simulink model "Copy_of_AUV_main"  (R2020b)
settings: Solver=VariableStepAuto  StartTime=0.0  StopTime=400  FixedStep=0.1  RelTol=1e-3
libraries: pid_lib x4, robotcorelib x2, dspsigops x1
settings Model: Creator=shanerutherford  LastModifiedBy=shanerutherford
settings SolverCC: ZeroCrossAlgorithm=Adaptive
settings DebuggingCC: IgnoredZcDiagnostic=none

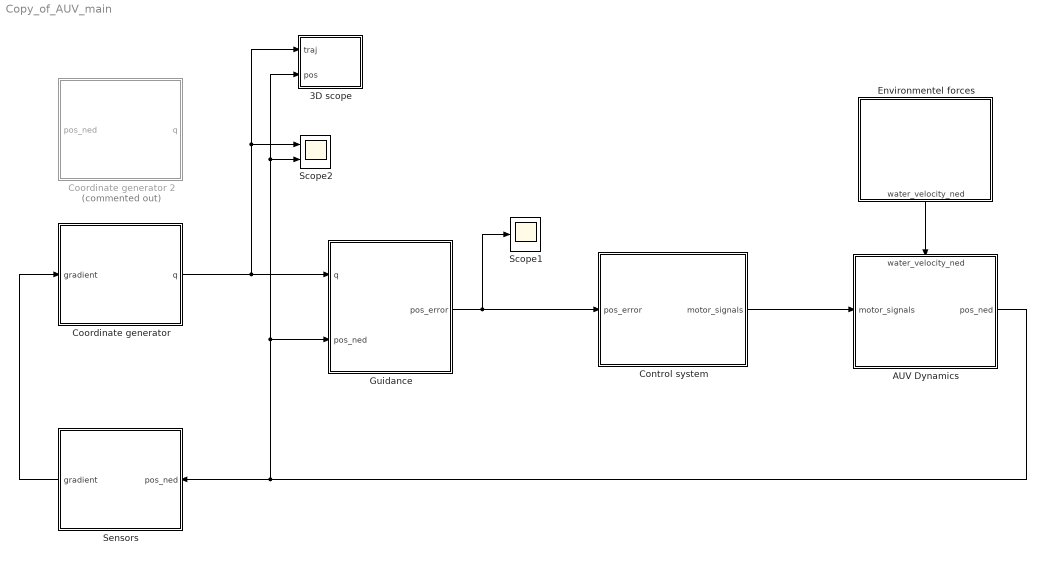
== system Copy_of_AUV_main ==
  3D scope : Subsystem
  AUV Dynamics : Subsystem
      settings: PortSchema="{\"entries\":[{\"content\":{\"sides\":[{\"content\":{\"connectorIds\":[\"In1\"]},\"type\":\"ConnectorPlacement.EquallySpacedRectSide\",\"uuid\":\"9ee444f3-b955-488d-8e49-640ea0f7df37\"},{\"content\":{\"connectorIds\":[\"Out1\"],\"side\":\"RIGHT\"},\"type\":\"ConnectorPlacement.EquallySpacedRectSide\",\"uuid\":\"ce4b5243-31e8-415d-aaa8-03cbb0c8065f\"},{\"content\":{\"connectorIds\":[\"In2\"],\"side\":\"TOP\"},\"type\":\"ConnectorPlacement.EquallySpacedRectSide\",\"uuid\":\"f69ed04b-67fd-4237-ab1a-d9f9564e83a0\"},{\"content\":{\"connectorIds\":[],\"side\":\"HIDDEN\"},\"type\":\"ConnectorPlacement.EquallySpacedRectSide\",\"uuid\":\"5b6b6d1e-b1c4-449c-9873-97d05fa29e3c\"}]},\"type\":\"ConnectorPlacement.EquallySpacedConnector\",\"uuid\":\"e4d51cd1-1a50-495c-8222-c38a5b01ba84\"}],\"packageUris\":[\"http://schema.mathworks.com/mf0/Connector/R2020b\"],\"version\":\"1.0\"}"
  Control system : Subsystem
  Coordinate generator : Subsystem
  Coordinate generator 2 : Subsystem  Commented=on
  Environmentel forces : Subsystem
      settings: PortSchema="{\"entries\":[{\"content\":{\"sides\":[{\"content\":{\"connectorIds\":[]},\"type\":\"ConnectorPlacement.EquallySpacedRectSide\",\"uuid\":\"0dd98e89-aff4-433c-b28f-c29455b8a07d\"},{\"content\":{\"connectorIds\":[],\"side\":\"RIGHT\"},\"type\":\"ConnectorPlacement.EquallySpacedRectSide\",\"uuid\":\"953662a4-5b51-4456-b69c-eca28c97a39b\"},{\"content\":{\"connectorIds\":[],\"side\":\"TOP\"},\"type\":\"ConnectorPlacement.EquallySpacedRectSide\",\"uuid\":\"911274c2-620a-4054-9b06-c69233cda7b5\"},{\"content\":{\"connectorIds\":[\"Out1\"],\"side\":\"BOTTOM\"},\"type\":\"ConnectorPlacement.EquallySpacedRectSide\",\"uuid\":\"d1098ec8-c176-4eae-9d99-8b466f13cb7d\"},{\"content\":{\"connectorIds\":[],\"side\":\"HIDDEN\"},\"type\":\"ConnectorPlacement.EquallySpacedRectSide\",\"uuid\":\"331d0c74-f854-4ce9-a20e-6d7219b69b25\"}]},\"type\":\"ConnectorPlacement.EquallySpacedConnector\",\"uuid\":\"51f6c218-3b35-4d9f-b9df-5dfda31bafc0\"}],\"packageUris\":[\"http://schema.mathworks.com/mf0/Connector/R2020b\"],\"version\":\"1.0\"}"
  Guidance : Subsystem
  Scope1 : Scope
  Scope2 : Scope  NumInputPorts=2
  Sensors : Subsystem
  wires:
  Guidance/1(pos_error) -> Control system/1(pos_error), Scope1/1
  AUV Dynamics/1(pos_ned) -> Sensors/1(pos_ned), 3D scope/2(pos), Scope2/2, Guidance/2(pos_ned)
  Environmentel forces/1(water_velocity_ned) -> AUV Dynamics/2(water_velocity_ned)
  Control system/1(motor_signals) -> AUV Dynamics/1(motor_signals)
  Coordinate generator/1(q) -> 3D scope/1(traj), Scope2/1, Guidance/1(q)
  Sensors/1(gradient) -> Coordinate generator/1(gradient)

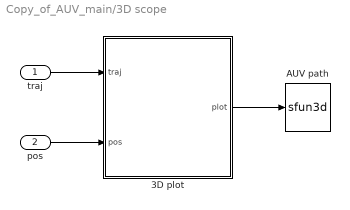
== system Copy_of_AUV_main/3D scope ==
  traj : Inport
  pos : Inport  Port=2
  3D plot : MATLAB Function  TreatAsAtomicUnit=on
  AUV path : S-Function  LoadFcn=if exist('sfun3d','file'), sfun3d([],[],[],'LoadBlock'); end  FunctionName=sfun3d  Parameters=ax,T,np,cp,gd,ls,mk,mx,hd,tb  SFunctionDeploymentMode=off  EnableBusSupport=off  mask(3D Graph){np=2, ax=[-15 15 -15 15 -20 20], mx=1e4, T=-1, cp=[0, 0 15], gd=on, hd=on, tb=on, ls=-, mk=none}
      mask prompts: np "Number of moving points (lines)"; ax "Range: [xmin xmax  ymin ymax zmin zmax]"; mx "Max number of points in each line"; T "Sampling Time"; cp "Camera position (use [0 0 1] for 2D XY view)"; gd "Grid (on|off)"; hd "HeadMarkers (on|off)"; tb "Toolbar (on|off)"; ls "LineStyle"; mk "LineMarker"
      mask help:
      | This block plots the position of several points in the XYZ space. The input contains the coordinates of all the points (x1,y1,z1,x2,y2,z2,...).
      | The number of moving points (lines), the XYZ ranges, sampling time, camera position, and grid (among other things) can be set as mask parameters.
      settings: CopyFcn=if exist('sfun3d','file'), sfun3d([],[],[],'CopyBlock'); end  DeleteFcn=if exist('sfun3d','file'), sfun3d([],[],[],'DeleteBlock'); end  NameChangeFcn=if exist('sfun3d','file'), sfun3d([],[],[],'NameChange'); end
      mask Help:
      | This block plots the position of several points in the XYZ space. The input contains the coordinates of all the points (x1,y1,z1,x2,y2,z2,...).
      | The number of moving points (lines), the XYZ ranges, sampling time, camera position, and grid (among other things) can be set as mask parameters.
      mask TypeOptions ls: - | -- | : | -. | none
      mask TypeOptions mk: none | . | + | o | * | x | square | diamond | v | ^ | > | < | pentagram | hexagram
      mask Display: plot([.05 .95 .95 .05 .05],[.45 .45 .95 .95 .45], 0.5+cos(0:0.1:2*pi)*0.3,0.7+sin(0:0.1:2*pi)*0.2)
  wires:
  3D plot/1(plot) -> AUV path/1
  traj/1 -> 3D plot/1(traj)
  pos/1 -> 3D plot/2(pos)

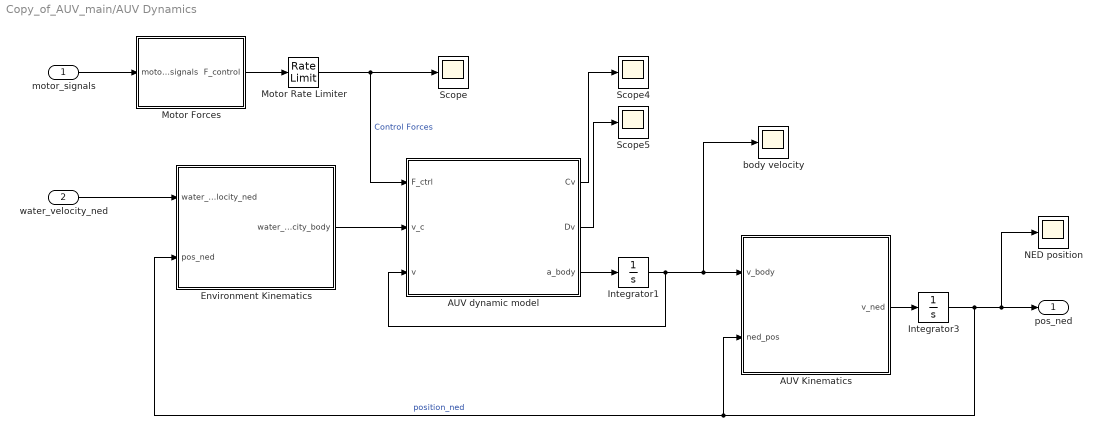
== system Copy_of_AUV_main/AUV Dynamics ==
  motor_signals : Inport
  water_velocity_ned : Inport  Port=2
  AUV Kinematics : MATLAB Function  TreatAsAtomicUnit=on
  AUV dynamic model : MATLAB Function  TreatAsAtomicUnit=on
  Environment Kinematics : MATLAB Function  TreatAsAtomicUnit=on
  Integrator1 : Integrator
  Integrator3 : Integrator
  Motor Forces : MATLAB Function  TreatAsAtomicUnit=on
  Motor Rate Limiter : RateLimiter  RisingSlewLimit=10  FallingSlewLimit=-10  SampleTimeMode=inherited
  NED position : Scope
  Scope : Scope
  Scope4 : Scope
  Scope5 : Scope
  body velocity : Scope
  pos_ned : Outport  PortDimensions=6
  wires:
  Integrator3/1 -> pos_ned/1, NED position/1, Environment Kinematics/2(pos_ned), AUV Kinematics/2(ned_pos)  "position_ned"
  Environment Kinematics/1(water_velocity_body) -> AUV dynamic model/2(v_c)
  AUV dynamic model/3(a_body) -> Integrator1/1
  AUV Kinematics/1(v_ned) -> Integrator3/1
  AUV dynamic model/1(Cv) -> Scope4/1
  Integrator1/1 -> AUV Kinematics/1(v_body), body velocity/1, AUV dynamic model/3(v)
  AUV dynamic model/2(Dv) -> Scope5/1
  water_velocity_ned/1 -> Environment Kinematics/1(water_velocity_ned)
  Motor Forces/1(F_control) -> Motor Rate Limiter/1
  motor_signals/1 -> Motor Forces/1(motor_signals)
  Motor Rate Limiter/1 -> AUV dynamic model/1(F_ctrl), Scope/1  "Control Forces"

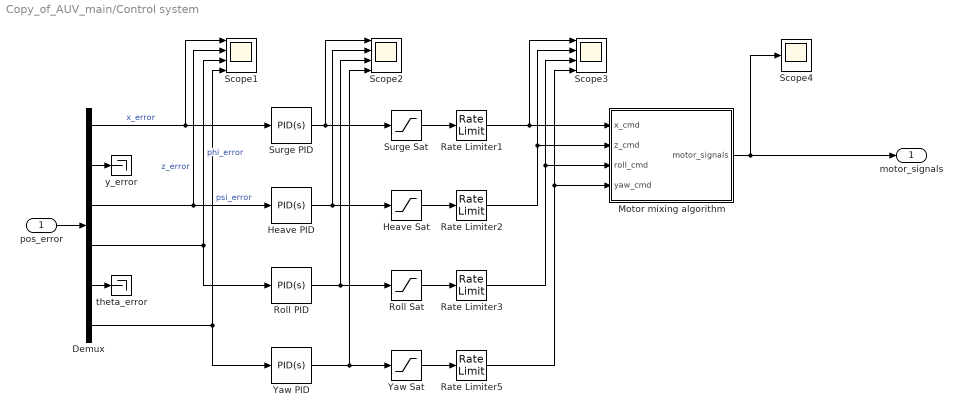
== system Copy_of_AUV_main/Control system ==
  pos_error : Inport
  Demux : Demux  Outputs=6
  Heave PID : pid_lib/PID Controller  Controller=PID  Form=Parallel  TimeDomain=Continuous-time  UseExternalTs=off  SampleTime=-1  IntegratorMethod=Forward Euler  FilterMethod=Forward Euler  ControllerParametersSource=internal  P=10  I=0  D=5  UseFilter=on  N=100  TunerSelectOption=Transfer Function Based (PID Tuner App)  InitialConditionSource=internal  InitialConditionForIntegrator=0  InitialConditionForFilter=0  DifferentiatorICPrevScaledInput=0  ExternalReset=none  TrackingMode=off  Kt=1  LimitOutput=on  SatLimitsSource=internal  UpperSaturationLimit=100  LowerSaturationLimit=-100  LinearizeAsGain=on  AntiWindupMode=none  Kb=1  POutMin=[]  POutMax=[]  IOutMin=[]  IOutMax=[]  DOutMin=[]  DOutMax=[]  NOutMin=[]  NOutMax=[]  SumOutMin=[]  SumOutMax=[]  SaturationOutMin=[]  SaturationOutMax=[]  PParamMin=[]  PParamMax=[]  IParamMin=[]  IParamMax=[]  DParamMin=[]  DParamMax=[]  NParamMin=[]  NParamMax=[]  KbParamMin=[]  KbParamMax=[]  KtParamMin=[]  KtParamMax=[]  KbOutMin=[]  KbOutMax=[]  KtOutMin=[]  KtOutMax=[]  IntegratorOutMin=[]  IntegratorOutMax=[]  FilterOutMin=[]  FilterOutMax=[]  SumI1OutMin=[]  SumI1OutMax=[]  SumI2OutMin=[]  SumI2OutMax=[]  SumI3OutMin=[]  SumI3OutMax=[]  SumI4OutMin=[]  SumI4OutMax=[]  SumDOutMin=[]  SumDOutMax=[]  DifferentiatorOutMin=[]  DifferentiatorOutMax=[]  FilterDiffOutCoefMin=[]  FilterDiffOutCoefMax=[]  ReciprocalOutMin=[]  ReciprocalOutMax=[]  SumDenOutMin=[]  SumDenOutMax=[]  SumNumOutMin=[]  SumNumOutMax=[]  DivideOutMin=[]  DivideOutMax=[]  UdiffTsProdOutMin=[]  UdiffTsProdOutMax=[]  NTsProdOutMin=[]  NTsProdOutMax=[]  UintegralTsProdOutMin=[]  UintegralTsProdOutMax=[]  UngainTsProdOutMin=[]  UngainTsProdOutMax=[]  IntegratorContinuousStateAttributes=''  IntegratorStateMustResolveToSignalObject=off  IntegratorRTWStateStorageClass=Auto  FilterContinuousStateAttributes=''  FilterStateMustResolveToSignalObject=off  FilterRTWStateStorageClass=Auto  ParallelPVariant=InternalParameters  IdealPVariant=Disabled  IVariant=InternalParameters  DVariant=InternalParameters  IntegratorVariant=Continuous  SatVariant=Enabled  AWVariant=Passthrough  PCopyVariant=Disabled  TRVariant=Disabled  FdbkBlocksVariant=Forward  IdealPFdbkVariant=Disabled  SatFdbkVariant=Disabled  DerivativeFilterVariant=ContFilter  NVariant=InternalParameters  NCopyVariant=Disabled  FilterICVariant=InternalICsFilter  IntegratorICVariant=InternalICs  ExternalResetVariant=Disabled  TRSumVariant=Passthrough  SumFdbkVariant=Disabled  SumVariant=Sum_PID  TsampFilterVariant=InternalTs  TsampNgainVariant=Passthrough  TsampIntegralVariant=Passthrough  ExternalSaturationOutDataTypeStr=Inherit: Same as second input
  Heave Sat : Saturate  UpperLimit=40  LowerLimit=-40  ZeroCross=off
  Motor mixing algorithm : MATLAB Function  TreatAsAtomicUnit=on
  Rate Limiter{1..3,5} (4 alike) : RateLimiter  RisingSlewLimit=20  FallingSlewLimit=-20  SampleTimeMode=inherited
  Roll PID : pid_lib/PID Controller  Controller=PID  Form=Parallel  TimeDomain=Continuous-time  UseExternalTs=off  SampleTime=-1  IntegratorMethod=Forward Euler  FilterMethod=Forward Euler  ControllerParametersSource=internal  P=20  I=0  D=10  UseFilter=on  N=100  TunerSelectOption=Transfer Function Based (PID Tuner App)  InitialConditionSource=internal  InitialConditionForIntegrator=0  InitialConditionForFilter=0  DifferentiatorICPrevScaledInput=0  ExternalReset=none  TrackingMode=off  Kt=1  LimitOutput=on  SatLimitsSource=internal  UpperSaturationLimit=100  LowerSaturationLimit=-100  LinearizeAsGain=on  AntiWindupMode=none  Kb=1  POutMin=[]  POutMax=[]  IOutMin=[]  IOutMax=[]  DOutMin=[]  DOutMax=[]  NOutMin=[]  NOutMax=[]  SumOutMin=[]  SumOutMax=[]  SaturationOutMin=[]  SaturationOutMax=[]  PParamMin=[]  PParamMax=[]  IParamMin=[]  IParamMax=[]  DParamMin=[]  DParamMax=[]  NParamMin=[]  NParamMax=[]  KbParamMin=[]  KbParamMax=[]  KtParamMin=[]  KtParamMax=[]  KbOutMin=[]  KbOutMax=[]  KtOutMin=[]  KtOutMax=[]  IntegratorOutMin=[]  IntegratorOutMax=[]  FilterOutMin=[]  FilterOutMax=[]  SumI1OutMin=[]  SumI1OutMax=[]  SumI2OutMin=[]  SumI2OutMax=[]  SumI3OutMin=[]  SumI3OutMax=[]  SumI4OutMin=[]  SumI4OutMax=[]  SumDOutMin=[]  SumDOutMax=[]  DifferentiatorOutMin=[]  DifferentiatorOutMax=[]  FilterDiffOutCoefMin=[]  FilterDiffOutCoefMax=[]  ReciprocalOutMin=[]  ReciprocalOutMax=[]  SumDenOutMin=[]  SumDenOutMax=[]  SumNumOutMin=[]  SumNumOutMax=[]  DivideOutMin=[]  DivideOutMax=[]  UdiffTsProdOutMin=[]  UdiffTsProdOutMax=[]  NTsProdOutMin=[]  NTsProdOutMax=[]  UintegralTsProdOutMin=[]  UintegralTsProdOutMax=[]  UngainTsProdOutMin=[]  UngainTsProdOutMax=[]  IntegratorContinuousStateAttributes=''  IntegratorStateMustResolveToSignalObject=off  IntegratorRTWStateStorageClass=Auto  FilterContinuousStateAttributes=''  FilterStateMustResolveToSignalObject=off  FilterRTWStateStorageClass=Auto  ParallelPVariant=InternalParameters  IdealPVariant=Disabled  IVariant=InternalParameters  DVariant=InternalParameters  IntegratorVariant=Continuous  SatVariant=Enabled  AWVariant=Passthrough  PCopyVariant=Disabled  TRVariant=Disabled  FdbkBlocksVariant=Forward  IdealPFdbkVariant=Disabled  SatFdbkVariant=Disabled  DerivativeFilterVariant=ContFilter  NVariant=InternalParameters  NCopyVariant=Disabled  FilterICVariant=InternalICsFilter  IntegratorICVariant=InternalICs  ExternalResetVariant=Disabled  TRSumVariant=Passthrough  SumFdbkVariant=Disabled  SumVariant=Sum_PID  TsampFilterVariant=InternalTs  TsampNgainVariant=Passthrough  TsampIntegralVariant=Passthrough  ExternalSaturationOutDataTypeStr=Inherit: Same as second input
  Roll Sat : Saturate  UpperLimit=40  LowerLimit=-40  ZeroCross=off
  Scope1 : Scope  NumInputPorts=4
  Scope2 : Scope  NumInputPorts=4
  Scope3 : Scope  NumInputPorts=4
  Scope4 : Scope
  Surge PID : pid_lib/PID Controller  Controller=PID  Form=Parallel  TimeDomain=Continuous-time  UseExternalTs=off  SampleTime=-1  IntegratorMethod=Forward Euler  FilterMethod=Forward Euler  ControllerParametersSource=internal  P=10  I=0  D=5  UseFilter=on  N=100  TunerSelectOption=Transfer Function Based (PID Tuner App)  InitialConditionSource=internal  InitialConditionForIntegrator=0  InitialConditionForFilter=0  DifferentiatorICPrevScaledInput=0  ExternalReset=none  TrackingMode=off  Kt=1  LimitOutput=on  SatLimitsSource=internal  UpperSaturationLimit=100  LowerSaturationLimit=-100  LinearizeAsGain=on  AntiWindupMode=none  Kb=1  POutMin=[]  POutMax=[]  IOutMin=[]  IOutMax=[]  DOutMin=[]  DOutMax=[]  NOutMin=[]  NOutMax=[]  SumOutMin=[]  SumOutMax=[]  SaturationOutMin=[]  SaturationOutMax=[]  PParamMin=[]  PParamMax=[]  IParamMin=[]  IParamMax=[]  DParamMin=[]  DParamMax=[]  NParamMin=[]  NParamMax=[]  KbParamMin=[]  KbParamMax=[]  KtParamMin=[]  KtParamMax=[]  KbOutMin=[]  KbOutMax=[]  KtOutMin=[]  KtOutMax=[]  IntegratorOutMin=[]  IntegratorOutMax=[]  FilterOutMin=[]  FilterOutMax=[]  SumI1OutMin=[]  SumI1OutMax=[]  SumI2OutMin=[]  SumI2OutMax=[]  SumI3OutMin=[]  SumI3OutMax=[]  SumI4OutMin=[]  SumI4OutMax=[]  SumDOutMin=[]  SumDOutMax=[]  DifferentiatorOutMin=[]  DifferentiatorOutMax=[]  FilterDiffOutCoefMin=[]  FilterDiffOutCoefMax=[]  ReciprocalOutMin=[]  ReciprocalOutMax=[]  SumDenOutMin=[]  SumDenOutMax=[]  SumNumOutMin=[]  SumNumOutMax=[]  DivideOutMin=[]  DivideOutMax=[]  UdiffTsProdOutMin=[]  UdiffTsProdOutMax=[]  NTsProdOutMin=[]  NTsProdOutMax=[]  UintegralTsProdOutMin=[]  UintegralTsProdOutMax=[]  UngainTsProdOutMin=[]  UngainTsProdOutMax=[]  IntegratorContinuousStateAttributes=''  IntegratorStateMustResolveToSignalObject=off  IntegratorRTWStateStorageClass=Auto  FilterContinuousStateAttributes=''  FilterStateMustResolveToSignalObject=off  FilterRTWStateStorageClass=Auto  ParallelPVariant=InternalParameters  IdealPVariant=Disabled  IVariant=InternalParameters  DVariant=InternalParameters  IntegratorVariant=Continuous  SatVariant=Enabled  AWVariant=Passthrough  PCopyVariant=Disabled  TRVariant=Disabled  FdbkBlocksVariant=Forward  IdealPFdbkVariant=Disabled  SatFdbkVariant=Disabled  DerivativeFilterVariant=ContFilter  NVariant=InternalParameters  NCopyVariant=Disabled  FilterICVariant=InternalICsFilter  IntegratorICVariant=InternalICs  ExternalResetVariant=Disabled  TRSumVariant=Passthrough  SumFdbkVariant=Disabled  SumVariant=Sum_PID  TsampFilterVariant=InternalTs  TsampNgainVariant=Passthrough  TsampIntegralVariant=Passthrough  ExternalSaturationOutDataTypeStr=Inherit: Same as second input
  Surge Sat : Saturate  UpperLimit=40  LowerLimit=-40  ZeroCross=off
  Yaw PID : pid_lib/PID Controller  Controller=PID  Form=Parallel  TimeDomain=Continuous-time  UseExternalTs=off  SampleTime=-1  IntegratorMethod=Forward Euler  FilterMethod=Forward Euler  ControllerParametersSource=internal  P=20  I=0  D=10  UseFilter=on  N=100  TunerSelectOption=Transfer Function Based (PID Tuner App)  InitialConditionSource=internal  InitialConditionForIntegrator=0  InitialConditionForFilter=0  DifferentiatorICPrevScaledInput=0  ExternalReset=none  TrackingMode=off  Kt=1  LimitOutput=on  SatLimitsSource=internal  UpperSaturationLimit=100  LowerSaturationLimit=-100  LinearizeAsGain=on  AntiWindupMode=none  Kb=1  POutMin=[]  POutMax=[]  IOutMin=[]  IOutMax=[]  DOutMin=[]  DOutMax=[]  NOutMin=[]  NOutMax=[]  SumOutMin=[]  SumOutMax=[]  SaturationOutMin=[]  SaturationOutMax=[]  PParamMin=[]  PParamMax=[]  IParamMin=[]  IParamMax=[]  DParamMin=[]  DParamMax=[]  NParamMin=[]  NParamMax=[]  KbParamMin=[]  KbParamMax=[]  KtParamMin=[]  KtParamMax=[]  KbOutMin=[]  KbOutMax=[]  KtOutMin=[]  KtOutMax=[]  IntegratorOutMin=[]  IntegratorOutMax=[]  FilterOutMin=[]  FilterOutMax=[]  SumI1OutMin=[]  SumI1OutMax=[]  SumI2OutMin=[]  SumI2OutMax=[]  SumI3OutMin=[]  SumI3OutMax=[]  SumI4OutMin=[]  SumI4OutMax=[]  SumDOutMin=[]  SumDOutMax=[]  DifferentiatorOutMin=[]  DifferentiatorOutMax=[]  FilterDiffOutCoefMin=[]  FilterDiffOutCoefMax=[]  ReciprocalOutMin=[]  ReciprocalOutMax=[]  SumDenOutMin=[]  SumDenOutMax=[]  SumNumOutMin=[]  SumNumOutMax=[]  DivideOutMin=[]  DivideOutMax=[]  UdiffTsProdOutMin=[]  UdiffTsProdOutMax=[]  NTsProdOutMin=[]  NTsProdOutMax=[]  UintegralTsProdOutMin=[]  UintegralTsProdOutMax=[]  UngainTsProdOutMin=[]  UngainTsProdOutMax=[]  IntegratorContinuousStateAttributes=''  IntegratorStateMustResolveToSignalObject=off  IntegratorRTWStateStorageClass=Auto  FilterContinuousStateAttributes=''  FilterStateMustResolveToSignalObject=off  FilterRTWStateStorageClass=Auto  ParallelPVariant=InternalParameters  IdealPVariant=Disabled  IVariant=InternalParameters  DVariant=InternalParameters  IntegratorVariant=Continuous  SatVariant=Enabled  AWVariant=Passthrough  PCopyVariant=Disabled  TRVariant=Disabled  FdbkBlocksVariant=Forward  IdealPFdbkVariant=Disabled  SatFdbkVariant=Disabled  DerivativeFilterVariant=ContFilter  NVariant=InternalParameters  NCopyVariant=Disabled  FilterICVariant=InternalICsFilter  IntegratorICVariant=InternalICs  ExternalResetVariant=Disabled  TRSumVariant=Passthrough  SumFdbkVariant=Disabled  SumVariant=Sum_PID  TsampFilterVariant=InternalTs  TsampNgainVariant=Passthrough  TsampIntegralVariant=Passthrough  ExternalSaturationOutDataTypeStr=Inherit: Same as second input
  Yaw Sat : Saturate  UpperLimit=40  LowerLimit=-40  ZeroCross=off
  theta_error : Terminator
  y_error : Terminator
  motor_signals : Outport
  wires:
  Demux/4 -> Scope1/3, Roll PID/1  "phi_error"
  Surge Sat/1 -> Rate Limiter1/1
  Demux/3 -> Scope1/2, Heave PID/1  "z_error"
  Roll Sat/1 -> Rate Limiter3/1
  Demux/6 -> Scope1/4, Yaw PID/1  "psi_error"
  Yaw Sat/1 -> Rate Limiter5/1
  Heave Sat/1 -> Rate Limiter2/1
  Demux/1 -> Scope1/1, Surge PID/1  "x_error"
  pos_error/1 -> Demux/1
  Demux/5 -> theta_error/1
  Demux/2 -> y_error/1
  Yaw PID/1 -> Scope2/4, Yaw Sat/1
  Roll PID/1 -> Roll Sat/1, Scope2/3
  Heave PID/1 -> Heave Sat/1, Scope2/2
  Surge PID/1 -> Surge Sat/1, Scope2/1
  Rate Limiter1/1 -> Scope3/1, Motor mixing algorithm/1(x_cmd)
  Rate Limiter2/1 -> Scope3/2, Motor mixing algorithm/2(z_cmd)
  Rate Limiter5/1 -> Motor mixing algorithm/4(yaw_cmd), Scope3/4
  Rate Limiter3/1 -> Scope3/3, Motor mixing algorithm/3(roll_cmd)
  Motor mixing algorithm/1(motor_signals) -> motor_signals/1, Scope4/1

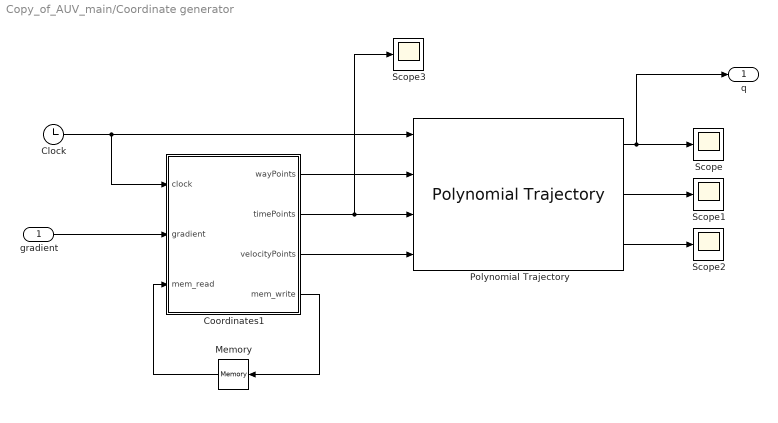
== system Copy_of_AUV_main/Coordinate generator ==
  gradient : Inport
  Clock : Clock
  Coordinates1 : MATLAB Function  TreatAsAtomicUnit=on
  Memory : Memory  InitialCondition=zeros(7, 5)
  Polynomial Trajectory : robotcorelib/Polynomial Trajectory  WaypointSource=External  Waypoints=[ 0, 2, 1, 5, 0; -1, 3, 1, 4, 4 ]  TimePoints=[ 0, 1, 2, 3, 4 ]  TimeInterval=[ 1, 4 ]  Method=Cubic Polynomial  ParameterSource=External  VelocityBoundaryCondition=zeros( 2, 5 )  AccelerationBoundaryCondition=zeros( 2, 5 )  SimulateUsing=Interpreted execution
  Scope{,1..3} (4 alike) : Scope
  q : Outport
  wires:
  Coordinates1/4(mem_write) -> Memory/1
  Polynomial Trajectory/3 -> Scope2/1
  Coordinates1/2(timePoints) -> Scope3/1, Polynomial Trajectory/3
  Coordinates1/3(velocityPoints) -> Polynomial Trajectory/4
  Clock/1 -> Coordinates1/1(clock), Polynomial Trajectory/1
  Coordinates1/1(wayPoints) -> Polynomial Trajectory/2
  Memory/1 -> Coordinates1/3(mem_read)
  Polynomial Trajectory/2 -> Scope1/1
  gradient/1 -> Coordinates1/2(gradient)
  Polynomial Trajectory/1 -> q/1, Scope/1

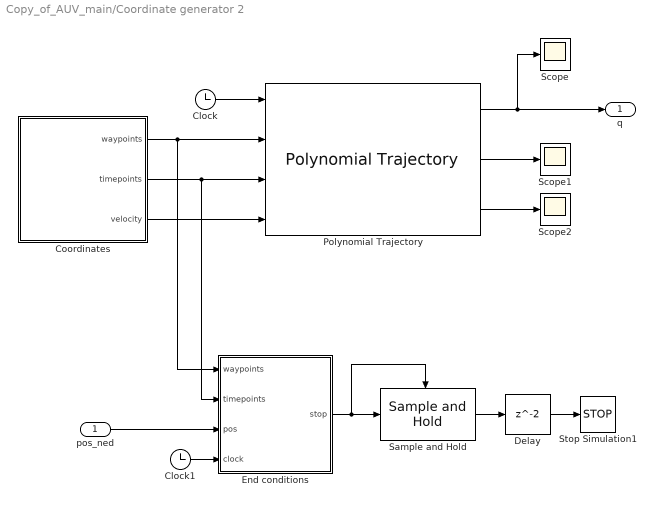
== system Copy_of_AUV_main/Coordinate generator 2 ==
  pos_ned : Inport
  Clock : Clock
  Clock1 : Clock
  Coordinates : MATLAB Function  TreatAsAtomicUnit=on
  Delay : Delay  InputProcessing=Columns as channels (frame based)
  End conditions : MATLAB Function  TreatAsAtomicUnit=on
  Polynomial Trajectory : robotcorelib/Polynomial Trajectory  WaypointSource=External  Waypoints=[ 0, 2, 1, 5, 0; -1, 3, 1, 4, 4 ]  TimePoints=[ 0, 1, 2, 3, 4 ]  TimeInterval=[ 1, 4 ]  Method=Cubic Polynomial  ParameterSource=External  VelocityBoundaryCondition=zeros( 2, 5 )  AccelerationBoundaryCondition=zeros( 2, 5 )  SimulateUsing=Interpreted execution
  Sample and Hold : dspsigops/Sample and Hold  trig=Rising edge  initCond=0  latchinput=off
  Scope : Scope
  Scope1 : Scope
  Scope2 : Scope
  Stop Simulation1 : Stop
  q : Outport
  wires:
  Coordinates/3(velocity) -> Polynomial Trajectory/4
  Polynomial Trajectory/1 -> Scope/1, q/1
  Polynomial Trajectory/3 -> Scope2/1
  Coordinates/2(timepoints) -> Polynomial Trajectory/3, End conditions/2(timepoints)
  Polynomial Trajectory/2 -> Scope1/1
  Coordinates/1(waypoints) -> Polynomial Trajectory/2, End conditions/1(waypoints)
  Clock/1 -> Polynomial Trajectory/1
  Clock1/1 -> End conditions/4(clock)
  pos_ned/1 -> End conditions/3(pos)
  Delay/1 -> Stop Simulation1/1
  End conditions/1(stop) -> Sample and Hold/Trigger, Sample and Hold/1
  Sample and Hold/1 -> Delay/1

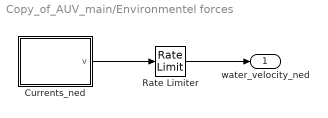
== system Copy_of_AUV_main/Environmentel forces ==
  Currents_ned : MATLAB Function  TreatAsAtomicUnit=on
  Rate Limiter : RateLimiter  RisingSlewLimit=10  FallingSlewLimit=-10  SampleTimeMode=inherited
  water_velocity_ned : Outport
  wires:
  Currents_ned/1(v) -> Rate Limiter/1
  Rate Limiter/1 -> water_velocity_ned/1

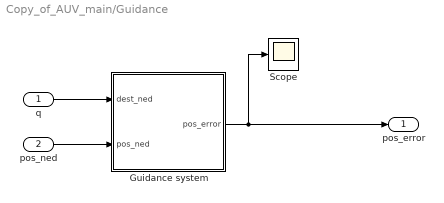
== system Copy_of_AUV_main/Guidance ==
  q : Inport
  pos_ned : Inport  Port=2
  Guidance system : MATLAB Function  TreatAsAtomicUnit=on
  Scope : Scope
  pos_error : Outport
  wires:
  q/1 -> Guidance system/1(dest_ned)
  Guidance system/1(pos_error) -> pos_error/1, Scope/1
  pos_ned/1 -> Guidance system/2(pos_ned)

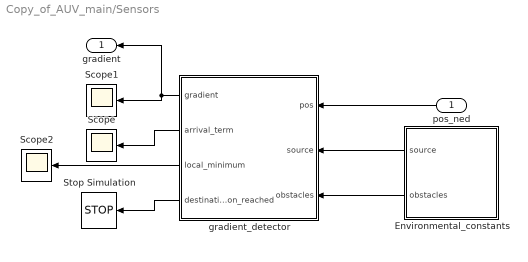
== system Copy_of_AUV_main/Sensors ==
  pos_ned : Inport
  Environmental_constants : MATLAB Function  TreatAsAtomicUnit=on
  Scope : Scope
  Scope1 : Scope
  Scope2 : Scope
  Stop Simulation : Stop
  gradient_detector : MATLAB Function  TreatAsAtomicUnit=on
  gradient : Outport
  wires:
  pos_ned/1 -> gradient_detector/1(pos)
  gradient_detector/1(gradient) -> Scope1/1, gradient/1
  gradient_detector/2(arrival_term) -> Scope/1
  Environmental_constants/1(source) -> gradient_detector/2(source)
  Environmental_constants/2(obstacles) -> gradient_detector/3(obstacles)
  gradient_detector/4(destination_reached) -> Stop Simulation/1
  gradient_detector/3(local_minimum) -> Scope2/1

== matlab function Copy_of_AUV_main/Coordinate generator 2/Coordinates ==
  data: waypoints output; timepoints output; velocity output
function [waypoints, timepoints, velocity] = fcn()

    avg_speed = 0.8; % m/s
    
    wp1 = [
        0,  5,   5,   5, -10,  -10, 0;
        0, 10, -10,  10,  10,  -10, 0;
        0,  0,   0,   0,   5,   10, 0; 
    ];

    wp2 = [
        0, 10, -10,  10, -10,  10, 0;
        0, 10,  10, -10, -10, -10, 0;
        0,  0,   5,  10,  10,  10, 0; 
    ];

    wp3 = [
        0, 10, 10, -10, -10,  10, -10, 0;
        0,  0, 10,  10,  10, -10,  10, 0;
        0,  0, 5,   10,   0,   0,   0, 0; 
    ];

    wp4 = [
        0, 10, 10, -10, -10,  10, 0;
        0,  0, 10,  10, -10, -10, 0;
        0,  0,  5,  10,  10,   5, 0;
    ];

    waypoints = wp2;
    
    [~, n] = size(waypoints);
    timepoints = zeros(1, n);
    for i = 2:n
        distance = norm(waypoints(1:3, i) - waypoints(1:3, i-1));
        timepoints(1, i) = timepoints(1, i-1) + distance/avg_speed;
    end
    
    velocity = zeros(size(waypoints));
    for i = 2:n-1
        vector = waypoints(1:3, i+1) - waypoints(1:3, i-1);
        if abs(sum(vector)) < 0.1
            w = waypoints(1:3, i) - waypoints(1:3, i-1);
            vector = [-w(2); w(1); 0];
        end
        unit_d = vector / norm(vector);
        velocity(1:3, i) = avg_speed * unit_d;
    end
end

== matlab function Copy_of_AUV_main/Control system/Motor mixing algorithm ==
  data: x_cmd input; motor_signals output size=[1, 4]; z_cmd input; roll_cmd input; yaw_cmd input
function motor_signals = fcn(x_cmd, z_cmd, roll_cmd, yaw_cmd)

motor_limit = 20;

if abs(x_cmd) + abs(yaw_cmd) > 2*motor_limit
    x_cmd = sign(x_cmd) * (2*motor_limit - abs(yaw_cmd));
end
if abs(z_cmd) + abs(roll_cmd) > 2*motor_limit
    z_cmd = sign(z_cmd) * (2*motor_limit - abs(roll_cmd));
end

front_right_motor = -0.5*z_cmd - 0.5*roll_cmd;
front_left_motor = -0.5*z_cmd + 0.5*roll_cmd;
back_right_motor = 0.5*x_cmd - 0.5*yaw_cmd;
back_left_motor = 0.5*x_cmd + 0.5*yaw_cmd;

motor_signals = [front_right_motor, front_left_motor, back_right_motor, back_left_motor];
end

== matlab function Copy_of_AUV_main/Sensors/Environmental_constants ==
  data: source output; obstacles output
function [source, obstacles] = fcn()

% Source that detector is looking for
source = [-6; 12; 8];

% obstacle to be avoided 
% coordinates ordered in top-left, top-right, bottom-right,  bottom-left
obstacles = [
    -5, 5, 5, -5; 
     5, 5, 5,  5; 
     10, 10, 0, 0
];

== matlab function Copy_of_AUV_main/3D scope/3D plot ==
  data: traj input; plot output; pos input
function plot = fcn(traj, pos)
 plot = [traj(2); traj(1); -traj(3); pos(2); pos(1); -pos(3)];

== matlab function Copy_of_AUV_main/Sensors/gradient_detector ==
  data: pos input; gradient output; arrival_term output; local_minimum output; source input; destination_reached output; obstacles input
function [gradient, arrival_term, local_minimum, destination_reached]= fcn(pos, source, obstacles)

    CONSIDER_OBSTACLES = 1;

    position = [pos(1); pos(2); pos(3)];

    % Calculate gradient due to obstacles
    
    % determine closest point on obstacle to position    
    if position(1) < obstacles(1, 4) && position(3) < obstacles(3, 4)
        % postion is to the bottom left of obstacle
        d_obs = obstacles(:, 4) - position;

    elseif position(1) < obstacles(1, 1) && position(3) > obstacles(3, 1)
        % postion is to the top left of obstacle
        d_obs = obstacles(:, 1) - position;

    elseif position(1) > obstacles(1, 3) && position(3) < obstacles(3, 3)
        % postion is to the bottom right of obstacle
        d_obs = obstacles(:, 3) - position;

    elseif position(1) > obstacles(1, 2) && position(3) > obstacles(3, 2)
        % postion is to the top right of obstacle
        d_obs = obstacles(:, 2) - position;

    elseif position(1) < obstacles(1, 1)
        % postion is to the left of obstacle
        d_obs = [obstacles(1,1) - position(1);
              obstacles(2,1) - position(2);
              0];
    elseif position(1) > obstacles(1, 2)
        % postion is to the right of obstacle
        d_obs = [obstacles(1, 2) - position(1);
              obstacles(2, 2) - position(2);
              0];
    elseif position(3) < obstacles(3, 3)
        % postion is below obsticle
        d_obs = [0;
              obstacles(2, 3) - position(2);
              obstacles(3, 3) - position(3)];
    elseif position(3) > obstacles(3, 2)
        % postion is above obstacle
        d_obs = [0;
              obstacles(2, 2) - position(2);
              obstacles(3, 2) - position(3)];
    else
        % position overlaps on y axis
        d_obs = [0;
              obstacles(2, 1) - position(2);
              0];
    end
    
    s1 = 0.5;         % Scaling factor which influences gradient attenuation
    Limit = 5;      % Set values to zero beyond this range
    
    if norm(d_obs) < Limit
        grad_obs = -s1/(s1+norm(d_obs)) * d_obs/norm(d_obs);
    else
        grad_obs = [0;0;0];
    end

    
    % Calculate gradient due to source
    s2 = 20;
    d_source = source - position;

    grad_source = (1 - s2/(s2+norm(d_source))) * d_source/norm(d_source);

    
    % Sum gradients together
    S_total = 5;    % Scaling factor
    if CONSIDER_OBSTACLES == 1
        gradient = S_total * (grad_source + grad_obs);
    else
        gradient = S_total * grad_source;
    end
    
    % Check if the AUV is stuck in a local minimum
    
    ang_diff = atan2(norm(cross(grad_source, grad_obs)), dot(grad_source, grad_obs)); % Angle between gradients
    mag_diff = norm((grad_source) + (grad_obs)); % Magnitude of gradients
    local_minimum = [ang_diff, mag_diff];
    
    % End simulation if source is very close
    destination_reached = 0;
    arrival_term = 1 - norm(grad_source);
    if arrival_term > 0.9
        destination_reached = 1;
    end
end

== matlab function Copy_of_AUV_main/Environmentel forces/Currents_ned ==
  data: v output
function v = fcn()
    % currents are irrotational
    v = [0; 0; 0];
end

== matlab function Copy_of_AUV_main/AUV Dynamics/Motor Forces ==
  data: F_control output size=6; motor_signals input
function F_control = fcn(motor_signals)
% x, y and z axis relates to local front (bow), starboard and down
% directions
% phi, theta and psi represents roll, pitch and yaw respectivly

% assuming that the force produced by each motor is proportonal to the
% signal voltage

thrust_constant = 1;
roll_constant = 1;
yaw_constant = 1;

FrontRight_m = motor_signals(1);
FrontLeft_m = motor_signals(2);
BackRight_m = motor_signals(3);
BackLeft_m = motor_signals(4);

F_control = [thrust_constant*(BackRight_m+BackLeft_m); 
      0;                                            % AUV cannot move in y direction
      -thrust_constant*(FrontRight_m+FrontLeft_m);  % positive z is downward 
      roll_constant*(FrontLeft_m-FrontRight_m);     % positive rotation is clockwise
      0;                                            % AUV cannot pitch 
      yaw_constant*(BackLeft_m-BackRight_m);
];

== matlab function Copy_of_AUV_main/AUV Dynamics/AUV Kinematics ==
  data: v_body input; ned_pos input; v_ned output
function v_ned = fcn(v_body, ned_pos)

% calculate Jacobian using MSS toolbox function
    [J, ~, ~] = eulerang(ned_pos(4), ned_pos(5), ned_pos(6)); 
    v_ned = J * v_body;
end

== matlab function Copy_of_AUV_main/Coordinate generator 2/End conditions ==
  data: waypoints input; timepoints input; pos input; clock input; stop output
function stop = fcn(waypoints, timepoints, pos, clock)

    final_n_error = abs(pos(1) - waypoints(1, end));
    final_e_error = abs(pos(2) - waypoints(2, end));
    final_d_error = abs(pos(3) - waypoints(3, end));
    final_pos_error = final_n_error + final_e_error + final_d_error;
    acceptance_radius = 0.5;

    if clock > timepoints(1, end) && final_pos_error < acceptance_radius
        stop = 1;
    else
        stop = 0;
    end
end

== matlab function Copy_of_AUV_main/AUV Dynamics/AUV dynamic model ==
  data: F_ctrl input; Cv output; Dv output; a_body output size=6; v_c input; v input
function [Cv, Dv, a_body] = fcn(F_ctrl, v_c, v)

v_r = v - v_c;
[M, C, D, g] = AUV_dynamic_model(v_r);    

% For output scope
Cv = C*v_r;
Dv = D*v_r;

a_body = M\(F_ctrl - C*v_r - D*v_r - g);

== matlab function Copy_of_AUV_main/Guidance/Guidance system ==
  data: dest_ned input; pos_error output; pos_ned input
function pos_error = fcn(dest_ned, pos_ned)
    % note that x is north, y is east and z is down    
    N_error = dest_ned(1)-pos_ned(1);
    E_error = dest_ned(2)-pos_ned(2);
    D_error = dest_ned(3)-pos_ned(3);

    current_heading = pos_ned(6);
    desired_heading = atan2(E_error, N_error);

    % convert to body axis
    x_error = max([-1, N_error*cos(current_heading)+E_error*sin(current_heading)]);
    y_error = 0;
    z_error = D_error;

    roll_error = 0;
    pitch_error = 0;
    yaw_error = desired_heading - current_heading;
    
    while roll_error > pi
        roll_error = roll_error - 2*pi;
    end
    while roll_error < -pi
        roll_error = roll_error + 2*pi;
    end

    while yaw_error > pi
        yaw_error = yaw_error - 2*pi;
    end
    while yaw_error < -pi
        yaw_error = yaw_error + 2*pi;
    end
    
    % Scale x_error down when yaw_error is high 
    k_angle = yaw_error*3;
    if k_angle > pi || k_angle < -pi
        k_angle = pi;
    end
     
    k = 0.5*cos(k_angle)+0.5;
    x_error = x_error*k;
    
    % Prevent turning if XY destination is nearby
%      arrival_error = 0.2;
%      NE_error = abs(N_error) + abs(E_error);
%      if NE_error < arrival_error
%          x_error = 0;
%          yaw_error = 0; % to prevent circling
%      end
%      if abs(D_error) < arrival_error
%          z_error = 0;
%      end
    
    pos_error = [x_error; y_error; z_error; roll_error; pitch_error; yaw_error];
end

== matlab function Copy_of_AUV_main/AUV Dynamics/Environment Kinematics ==
  data: water_velocity_ned input; water_velocity_body output size=6; pos_ned input
function water_velocity_body = fcn(water_velocity_ned, pos_ned)
    euler_ang = rotateZYX(pos_ned(4), pos_ned(5), pos_ned(6));
    w_v =  euler_ang * water_velocity_ned;
    water_velocity_body = [w_v(1); w_v(2); w_v(3); 0; 0; 0];
end

== matlab function Copy_of_AUV_main/Coordinate generator/Coordinates1 ==
  settings: updateMethod=DISCRETE  sampleTime=2
  data: wayPoints output; timePoints output; velocityPoints output; clock input; gradient input; mem_read input; mem_write output
function [wayPoints, timePoints, velocityPoints, mem_write] = fcn(clock, gradient, mem_read)

    % Calculate best waypoints for path generation

    avg_speed = 0.8; % m/s
    
    % Should run one time to initalise waypoints
    if mem_read == 0
        wayPoints = [
            zeros(3, 1), 0.1*gradient, 0.2*gradient, 0.3*gradient, 0.4*gradient;
        ];
        timePoints = ones(1, 5);
        timePoints(1, 1) = 0;
        velocityPoints = zeros(3, 5);
    else
        wayPoints = mem_read(1:3, 1:5);
        timePoints = mem_read(4, 1:5);
        velocityPoints = mem_read(5:7, 1:5);
    end
    
    
    % Enter a new waypoint and cycle waypoints
    [~, n] = size(wayPoints);
    if clock > timePoints(1, 4)
        for i = 1:n-1
            wayPoints(1:3, i) = wayPoints(1:3, i+1);
            timePoints(1, i) = timePoints(1, i+1);
            velocityPoints(1:3, i) = velocityPoints(1:3, i+1);
        end
        wayPoints(1:3, n) = wayPoints(1:3, n) + gradient;
    end


    
    % Generate timepoints
    for i = 2:n
        distance = norm(wayPoints(1:3, i) - wayPoints(1:3, i-1));
        if distance < 0.1
            % stop for a few seconds if distance is 0
            timePoints(1, i) = timePoints(1, i-1) + 1;
        else
            timePoints(1, i) = timePoints(1, i-1) + distance/avg_speed;
        end
    end
    
    % Generate velocity points
    for i = 2:n-1
        L_1_2 = wayPoints(1:3, i+1) - wayPoints(1:3, i);
        L_1_3 = wayPoints(1:3, i+1) - wayPoints(1:3, i-1);
        
        if abs(sum(L_1_2)) < 0.1        % if current point is same as next point
            unit_v = zeros(3, 1);       % stop
            
        elseif abs(sum(L_1_3)) < 0.1    % if previous point is same as next point
            % velocity direction is parallel to line connecting current point and previous point 
            w = wayPoints(1:3, i) - wayPoints(1:3, i-1);
            L_parallel = [-w(2); w(1); 0];
            unit_v = L_parallel / norm(L_parallel);
        else
            % Otherwise, velocity direction is parallel to line connecting
            % previous point and next point
            unit_v = L_1_3 / norm(L_1_3);
        end
        
        velocityPoints(1:3, i) = avg_speed*unit_v;
    end
    
    % Save data for next iteration
    mem_write = [
        wayPoints; 
        timePoints;
        velocityPoints];
end
